simulink model "sl_GDT_C_RRR"  (R2016b)
settings: Solver=ode45  StartTime=0.0  StopTime=5  MaxStep=1e-3  RelTol=1e-8  EnableMultiTasking=on
settings Model: ExtModeTrigMode=oneshot  ExtModeArmWhenConnect=off  Creator=Manuel G. Ortega  LastModifiedBy=marrcogrova
settings DataIOCC: SaveFormat=Array  SignalLoggingSaveFormat=ModelDataLogs
settings OptimizationCC: BooleanDataType=off  ExpressionDepthLimit=2147483647  InitFltsAndDblsToZero=on  LifeSpan=inf
settings DebuggingCC: SaveWithParameterizedLinksMsg=none  UnderspecifiedInitializationDetection=Classic  MergeDetectMultiDrivingBlocksExec=none  SignalResolutionControl=TryResolveAllWithWarning  MultiTaskDSMMsg=warning  MultiTaskCondExecSysMsg=none  FcnCallInpInsideContextMsg=warning  StateNameClashWarn=warning  SFUnexpectedBacktrackingDiag=warning  SFNoUnconditionalDefaultTransitionDiag=warning  SFExecutionAtInitializationDiag=none
settings HardwareCC: ProdBitPerPointer=32  ProdBitPerSizeT=32  ProdBitPerPtrDiffT=32  ProdLargestAtomicFloat=None  ProdIntDivRoundTo=Undefined  ProdEndianess=Unspecified  ProdWordSize=32  ProdHWDeviceType=32-bit Generic  TargetUnknown=on
settings ModelReferenceCC: PropagateSignalLabelsOutOfModel=off
settings GRTTargetCC: TargetFcnLib=ansi_tfl_tmw.mat  TargetLangStandard=C89/C90 (ANSI)  GeneratePreprocessorConditionals=Disable all  CombineOutputUpdateFcns=off  GRTInterface=on
settings ConfigComp: CovMetricSettings=dw  CovHtmlReporting=on  CovSaveCumulativeToWorkspaceVar=on  CovSaveSingleToWorkspaceVar=on  CovExternalEMLEnable=off  CovSFcnEnable=off

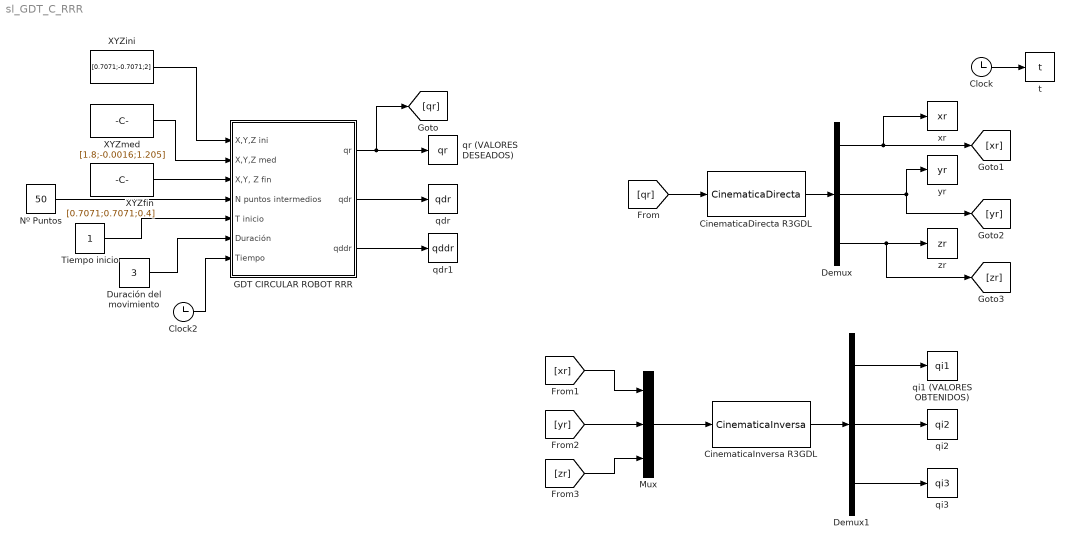
== system sl_GDT_C_RRR ==
  CinematicaDirecta R3GDL : MATLABFcn  MATLABFcn=CinematicaDirecta  OutputDimensions=3
  CinematicaInversa R3GDL : MATLABFcn  MATLABFcn=CinematicaInversa  OutputDimensions=3
  Clock : Clock
  Clock2 : Clock
  Demux : Demux  Outputs=3
  Demux1 : Demux  Outputs=3
  Duración del movimiento : Constant  Value=3
  GDT CIRCULAR ROBOT RRR : Subsystem
  Mux : Mux  Inputs=3
  Nº Puntos : Constant  Value=50
  Tiempo inicio : Constant
  XYZfin : Constant  Value=[0.7071;0.7071;0.4]
  XYZini : Constant  Value=[0.7071;-0.7071;2]
  XYZmed : Constant  Value=[1.8;-0.0016;1.205]
  qdr : ToWorkspace  VariableName=qdr  SampleTime=-1
  qdr1 : ToWorkspace  VariableName=qddr  SampleTime=-1
  qi1 (VALORES OBTENIDOS) : ToWorkspace  VariableName=qi1  SampleTime=-1
  "qi2 " : ToWorkspace  VariableName=qi2  SampleTime=-1
  "qi3 " : ToWorkspace  VariableName=qi3  SampleTime=-1
  qr (VALORES DESEADOS) : ToWorkspace  VariableName=qr  SampleTime=-1
  t : ToWorkspace  VariableName=t  SampleTime=-1
  xr : ToWorkspace  VariableName=xr  SampleTime=-1
  yr : ToWorkspace  VariableName=yr  SampleTime=-1
  zr : ToWorkspace  VariableName=zr  SampleTime=-1
  wires:
  Clock/1 -> t/1
  Clock2/1 -> GDT CIRCULAR ROBOT RRR/7(Tiempo)
  Duración del movimiento/1 -> GDT CIRCULAR ROBOT RRR/6(Duración)
  Tiempo inicio/1 -> GDT CIRCULAR ROBOT RRR/5(T inicio)
  Nº Puntos/1 -> GDT CIRCULAR ROBOT RRR/4(N puntos intermedios)
  XYZfin/1 -> GDT CIRCULAR ROBOT RRR/3("X,Y, Z fin")
  XYZini/1 -> GDT CIRCULAR ROBOT RRR/1(X,Y,Z ini)
  GDT CIRCULAR ROBOT RRR/1(qr) -> [qr], qr (VALORES DESEADOS)/1
  [qr] -> CinematicaDirecta R3GDL/1
  CinematicaDirecta R3GDL/1 -> Demux/1
  Demux/1 -> xr/1, [xr]
  Demux/2 -> [yr], yr/1
  Demux/3 -> [zr], zr/1
  [yr] -> Mux/2
  [zr] -> Mux/3
  [xr] -> Mux/1
  Mux/1 -> CinematicaInversa R3GDL/1
  CinematicaInversa R3GDL/1 -> Demux1/1
  Demux1/1 -> qi1 (VALORES OBTENIDOS)/1
  Demux1/3 -> "qi3 "/1
  Demux1/2 -> "qi2 "/1
  GDT CIRCULAR ROBOT RRR/2(qdr) -> qdr/1
  GDT CIRCULAR ROBOT RRR/3(qddr) -> qdr1/1
  XYZmed/1 -> GDT CIRCULAR ROBOT RRR/2("X,Y,Z med ")

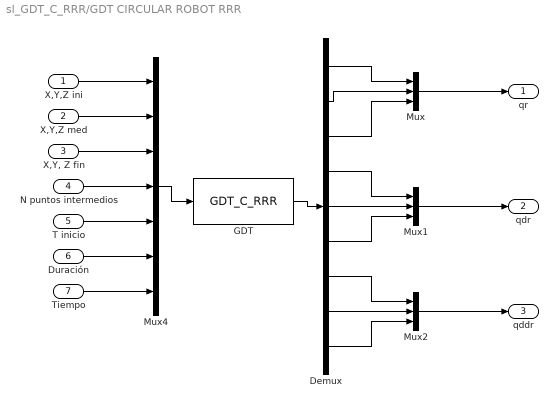
== system sl_GDT_C_RRR/GDT CIRCULAR ROBOT RRR ==
  X,Y,Z ini : Inport
  "X,Y,Z med " : Inport  Port=2
  "X,Y, Z fin" : Inport  Port=3
  N puntos intermedios : Inport  Port=4
  T inicio : Inport  Port=5
  Duración : Inport  Port=6
  Tiempo : Inport  Port=7
  Demux : Demux  Outputs=9
  "GDT " : MATLABFcn  MATLABFcn=GDT_C_RRR  OutputDimensions=9
  Mux : Mux  Inputs=3
  Mux1 : Mux  Inputs=3
  Mux2 : Mux  Inputs=3
  Mux4 : Mux  Inputs=7
  qr : Outport
  qdr : Outport  Port=2
  qddr : Outport  Port=3
  wires:
  Mux4/1 -> "GDT "/1
  "GDT "/1 -> Demux/1
  Mux/1 -> qr/1
  Demux/1 -> Mux/1
  Demux/2 -> Mux/2
  Demux/3 -> Mux/3
  Demux/5 -> Mux1/2
  Demux/4 -> Mux1/1
  Demux/6 -> Mux1/3
  Mux1/1 -> qdr/1
  Demux/8 -> Mux2/2
  Mux2/1 -> qddr/1
  Demux/7 -> Mux2/1
  Demux/9 -> Mux2/3
  X,Y,Z ini/1 -> Mux4/1
  "X,Y,Z med "/1 -> Mux4/2
  "X,Y, Z fin"/1 -> Mux4/3
  N puntos intermedios/1 -> Mux4/4
  T inicio/1 -> Mux4/5
  Duración/1 -> Mux4/6
  Tiempo/1 -> Mux4/7
